simulink model "AutomaticWateringSystemProject"  (R2013b)
settings: Solver=ode3  SolverMode=SingleTasking  StartTime=0.0  StopTime=10.0  RelTol=1e-3
PreLoadFcn:
  | waijung.modelPreload; % Required for working with Waijung Blockset. Do not remove.
undefined symbols (not defined in the file): HSEOSC, Link, LQFP100, ST, STM32F407VG
libraries: stm32f4_io_lib x6, stm32f4_adc_lib x1, stm32f4_device_config_lib x1
(part 2 of 2)

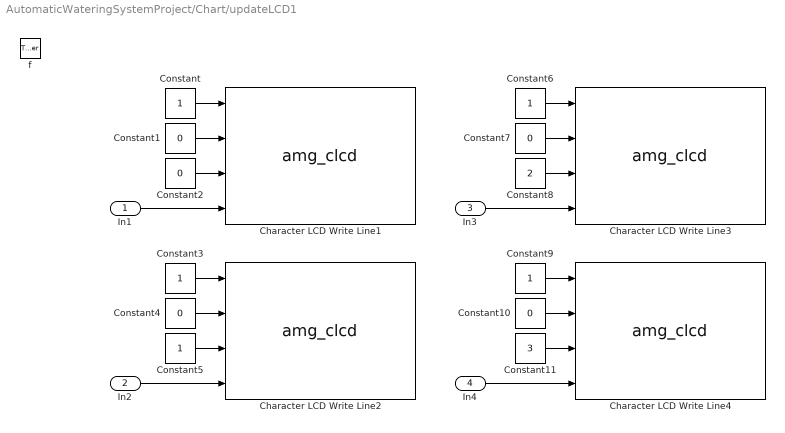
== system AutomaticWateringSystemProject/Chart/updateLCD1 ==
  In1 : Inport  OutDataTypeStr=uint8  PortDimensions=[1 16]
  In2 : Inport  Port=2  OutDataTypeStr=uint8  PortDimensions=[1 16]
  In3 : Inport  Port=3  OutDataTypeStr=uint8  PortDimensions=[1 16]
  In4 : Inport  Port=4  OutDataTypeStr=uint8  PortDimensions=[1 16]
  f : TriggerPort  TriggerType=function-call
      settings: CopyFcn=Stateflow.SLINSF.SimulinkMan.removeBlockPreDeleteFcn  PreDeleteFcn=Stateflow.SLINSF.SimulinkMan.unsafePredeleteFcn
  Character LCD Write Line1 : S-Function  FunctionName=amg_clcd  Parameters=module,configuration,inputtypearray,outputtypearray,confstr,sampletime,sampletimestr,blockid  EnableBusSupport=off  mask(amg_clcd){configuration=Transaction, module=1, model=amg CLCD Std, interface=4-bits, linecount=4, columncount=20, gpiotype=Push-pull, controlport=E, control_rs=15, control_rw=13, control_en=11, dataport=A, data0=7, data1=5, data2=3, data3=1, usestringbuffer=off, stringbuffer=<empty>, varname=, inputtypearray=[4 -1 -1 -1 -1], outputtypearray=[0], confstr=["4","4","20","PP","E","15","11","13","","A","","","","","7","5","3","1","0","","1","0","0","0","1","0","0","0","0","stm32f4"], sampletime=-1, sampletimestr=-1, blockid=ChartupdateLCD1CharacterLCDWriteLine1}
      mask prompts: model "LCD model:"; linecount "Number of lines:"; columncount "Number of columns:"; gpiotype "GPIO Output type:"; controlport "GPIO control port:"; control_rs "GPIO control pin, RS:"; control_rw "GPIO control pin, RW:"; control_en "GPIO control pin, EN:"; dataport "GPIO data D[7:4] port"; data0 "GPIO data pin, D4:"; data1 "GPIO data pin, D5:"; data2 "GPIO data pin, D6:"; data3 "GPIO data pin, D7:"; usestringbuffer "Use string buffer"; stringbuffer "String buffer"; varname "Variable name"; inputtypearray "Input type array"; outputtypearray "Output type array"; confstr "Configuration string"; sampletime "Sample time (sec)"; sampletimestr "Compiled sample time (sec) in string"
      mask help:
      | Note for cmd:
      | 1 - Clear specified LCD line display before write data to LCD.
      | Otherwise (e.g. 0) - Write data without clearing LCD Line.
      |
      | Position:
      | x = 0, First Character (from left to right)
      | y = 0, Top Line
      mask init:
      | amg_clcd_callback('init');
      mask Help: web(fullfile(waijungdocroot,'amg_clcd_write.htm'), '-browser')
      mask TypeOptions configuration: Setup | Transaction
      mask Callback configuration: amg_clcd_callback('configuration');
      mask TypeOptions module: 1 | 2 | 3 | 4
      mask TypeOptions model: amg CLCD Std
      mask TypeOptions interface: 4-bits
      mask TypeOptions gpiotype: Push-pull | Open-drain
      mask TypeOptions controlport: A | B | C | D | E | F | G | H | I
      mask TypeOptions control_rs: 0 | 1 | 2 | 3 | 4 | 5 | 6 | 7 | 8 | 9 | 10 | 11 | 12 | 13 | 14 | 15
      mask TypeOptions control_rw: 0 | 1 | 2 | 3 | 4 | 5 | 6 | 7 | 8 | 9 | 10 | 11 | 12 | 13 | 14 | 15
      mask TypeOptions control_en: 0 | 1 | 2 | 3 | 4 | 5 | 6 | 7 | 8 | 9 | 10 | 11 | 12 | 13 | 14 | 15
      mask TypeOptions dataport: A | B | C | D | E | F | G | H | I
      mask TypeOptions data0: 0 | 1 | 2 | 3 | 4 | 5 | 6 | 7 | 8 | 9 | 10 | 11 | 12 | 13 | 14 | 15
      mask TypeOptions data1: 0 | 1 | 2 | 3 | 4 | 5 | 6 | 7 | 8 | 9 | 10 | 11 | 12 | 13 | 14 | 15
      mask TypeOptions data2: 0 | 1 | 2 | 3 | 4 | 5 | 6 | 7 | 8 | 9 | 10 | 11 | 12 | 13 | 14 | 15
      mask TypeOptions data3: 0 | 1 | 2 | 3 | 4 | 5 | 6 | 7 | 8 | 9 | 10 | 11 | 12 | 13 | 14 | 15
      mask Callback usestringbuffer: amg_clcd_callback('usestringbuffer');
      mask TypeOptions stringbuffer: <empty>
      mask Callback varname: amg_clcd_callback('varname');
      mask Callback confstr: amg_clcd_callback('confstr');
      mask Callback sampletime: amg_clcd_callback('sampletime');
      mask Callback sampletimestr: amg_clcd_callback('sampletimestr');
      mask Callback blockid: amg_clcd_callback('blockid');
      mask Display: text(0.5, 0.5, 'Module: CLCD1 (Write)\nTs (sec): -1','ver','middle','hor','center');port_label('input', 1,'cmd');port_label('input', 2,'xpos');port_label('input', 3,'ypos');port_label('input', 4,'str');
  Character LCD Write Line2 : S-Function  FunctionName=amg_clcd  Parameters=module,configuration,inputtypearray,outputtypearray,confstr,sampletime,sampletimestr,blockid  EnableBusSupport=off  mask(amg_clcd){configuration=Transaction, module=1, model=amg CLCD Std, interface=4-bits, linecount=4, columncount=20, gpiotype=Push-pull, controlport=E, control_rs=15, control_rw=13, control_en=11, dataport=A, data0=7, data1=5, data2=3, data3=1, usestringbuffer=off, stringbuffer=<empty>, varname=, inputtypearray=[4 -1 -1 -1 -1], outputtypearray=[0], confstr=["4","4","20","PP","E","15","11","13","","A","","","","","7","5","3","1","0","","1","0","0","0","1","0","0","0","0","stm32f4"], sampletime=-1, sampletimestr=-1, blockid=ChartupdateLCD1CharacterLCDWriteLine2}
      mask prompts: model "LCD model:"; linecount "Number of lines:"; columncount "Number of columns:"; gpiotype "GPIO Output type:"; controlport "GPIO control port:"; control_rs "GPIO control pin, RS:"; control_rw "GPIO control pin, RW:"; control_en "GPIO control pin, EN:"; dataport "GPIO data D[7:4] port"; data0 "GPIO data pin, D4:"; data1 "GPIO data pin, D5:"; data2 "GPIO data pin, D6:"; data3 "GPIO data pin, D7:"; usestringbuffer "Use string buffer"; stringbuffer "String buffer"; varname "Variable name"; inputtypearray "Input type array"; outputtypearray "Output type array"; confstr "Configuration string"; sampletime "Sample time (sec)"; sampletimestr "Compiled sample time (sec) in string"
      mask help:
      | Note for cmd:
      | 1 - Clear specified LCD line display before write data to LCD.
      | Otherwise (e.g. 0) - Write data without clearing LCD Line.
      |
      | Position:
      | x = 0, First Character (from left to right)
      | y = 0, Top Line
      mask init:
      | amg_clcd_callback('init');
      mask Help: web(fullfile(waijungdocroot,'amg_clcd_write.htm'), '-browser')
      mask TypeOptions configuration: Setup | Transaction
      mask Callback configuration: amg_clcd_callback('configuration');
      mask TypeOptions module: 1 | 2 | 3 | 4
      mask TypeOptions model: amg CLCD Std
      mask TypeOptions interface: 4-bits
      mask TypeOptions gpiotype: Push-pull | Open-drain
      mask TypeOptions controlport: A | B | C | D | E | F | G | H | I
      mask TypeOptions control_rs: 0 | 1 | 2 | 3 | 4 | 5 | 6 | 7 | 8 | 9 | 10 | 11 | 12 | 13 | 14 | 15
      mask TypeOptions control_rw: 0 | 1 | 2 | 3 | 4 | 5 | 6 | 7 | 8 | 9 | 10 | 11 | 12 | 13 | 14 | 15
      mask TypeOptions control_en: 0 | 1 | 2 | 3 | 4 | 5 | 6 | 7 | 8 | 9 | 10 | 11 | 12 | 13 | 14 | 15
      mask TypeOptions dataport: A | B | C | D | E | F | G | H | I
      mask TypeOptions data0: 0 | 1 | 2 | 3 | 4 | 5 | 6 | 7 | 8 | 9 | 10 | 11 | 12 | 13 | 14 | 15
      mask TypeOptions data1: 0 | 1 | 2 | 3 | 4 | 5 | 6 | 7 | 8 | 9 | 10 | 11 | 12 | 13 | 14 | 15
      mask TypeOptions data2: 0 | 1 | 2 | 3 | 4 | 5 | 6 | 7 | 8 | 9 | 10 | 11 | 12 | 13 | 14 | 15
      mask TypeOptions data3: 0 | 1 | 2 | 3 | 4 | 5 | 6 | 7 | 8 | 9 | 10 | 11 | 12 | 13 | 14 | 15
      mask Callback usestringbuffer: amg_clcd_callback('usestringbuffer');
      mask TypeOptions stringbuffer: <empty>
      mask Callback varname: amg_clcd_callback('varname');
      mask Callback confstr: amg_clcd_callback('confstr');
      mask Callback sampletime: amg_clcd_callback('sampletime');
      mask Callback sampletimestr: amg_clcd_callback('sampletimestr');
      mask Callback blockid: amg_clcd_callback('blockid');
      mask Display: text(0.5, 0.5, 'Module: CLCD1 (Write)\nTs (sec): -1','ver','middle','hor','center');port_label('input', 1,'cmd');port_label('input', 2,'xpos');port_label('input', 3,'ypos');port_label('input', 4,'str');
  Character LCD Write Line3 : S-Function  FunctionName=amg_clcd  Parameters=module,configuration,inputtypearray,outputtypearray,confstr,sampletime,sampletimestr,blockid  EnableBusSupport=off  mask(amg_clcd){configuration=Transaction, module=1, model=amg CLCD Std, interface=4-bits, linecount=4, columncount=20, gpiotype=Push-pull, controlport=E, control_rs=15, control_rw=13, control_en=11, dataport=A, data0=7, data1=5, data2=3, data3=1, usestringbuffer=off, stringbuffer=<empty>, varname=, inputtypearray=[4 -1 -1 -1 -1], outputtypearray=[0], confstr=["4","4","20","PP","E","15","11","13","","A","","","","","7","5","3","1","0","","1","0","0","0","1","0","0","0","0","stm32f4"], sampletime=-1, sampletimestr=-1, blockid=ChartupdateLCD1CharacterLCDWriteLine3}
      mask prompts: model "LCD model:"; linecount "Number of lines:"; columncount "Number of columns:"; gpiotype "GPIO Output type:"; controlport "GPIO control port:"; control_rs "GPIO control pin, RS:"; control_rw "GPIO control pin, RW:"; control_en "GPIO control pin, EN:"; dataport "GPIO data D[7:4] port"; data0 "GPIO data pin, D4:"; data1 "GPIO data pin, D5:"; data2 "GPIO data pin, D6:"; data3 "GPIO data pin, D7:"; usestringbuffer "Use string buffer"; stringbuffer "String buffer"; varname "Variable name"; inputtypearray "Input type array"; outputtypearray "Output type array"; confstr "Configuration string"; sampletime "Sample time (sec)"; sampletimestr "Compiled sample time (sec) in string"
      mask help:
      | Note for cmd:
      | 1 - Clear specified LCD line display before write data to LCD.
      | Otherwise (e.g. 0) - Write data without clearing LCD Line.
      |
      | Position:
      | x = 0, First Character (from left to right)
      | y = 0, Top Line
      mask init:
      | amg_clcd_callback('init');
      mask Help: web(fullfile(waijungdocroot,'amg_clcd_write.htm'), '-browser')
      mask TypeOptions configuration: Setup | Transaction
      mask Callback configuration: amg_clcd_callback('configuration');
      mask TypeOptions module: 1 | 2 | 3 | 4
      mask TypeOptions model: amg CLCD Std
      mask TypeOptions interface: 4-bits
      mask TypeOptions gpiotype: Push-pull | Open-drain
      mask TypeOptions controlport: A | B | C | D | E | F | G | H | I
      mask TypeOptions control_rs: 0 | 1 | 2 | 3 | 4 | 5 | 6 | 7 | 8 | 9 | 10 | 11 | 12 | 13 | 14 | 15
      mask TypeOptions control_rw: 0 | 1 | 2 | 3 | 4 | 5 | 6 | 7 | 8 | 9 | 10 | 11 | 12 | 13 | 14 | 15
      mask TypeOptions control_en: 0 | 1 | 2 | 3 | 4 | 5 | 6 | 7 | 8 | 9 | 10 | 11 | 12 | 13 | 14 | 15
      mask TypeOptions dataport: A | B | C | D | E | F | G | H | I
      mask TypeOptions data0: 0 | 1 | 2 | 3 | 4 | 5 | 6 | 7 | 8 | 9 | 10 | 11 | 12 | 13 | 14 | 15
      mask TypeOptions data1: 0 | 1 | 2 | 3 | 4 | 5 | 6 | 7 | 8 | 9 | 10 | 11 | 12 | 13 | 14 | 15
      mask TypeOptions data2: 0 | 1 | 2 | 3 | 4 | 5 | 6 | 7 | 8 | 9 | 10 | 11 | 12 | 13 | 14 | 15
      mask TypeOptions data3: 0 | 1 | 2 | 3 | 4 | 5 | 6 | 7 | 8 | 9 | 10 | 11 | 12 | 13 | 14 | 15
      mask Callback usestringbuffer: amg_clcd_callback('usestringbuffer');
      mask TypeOptions stringbuffer: <empty>
      mask Callback varname: amg_clcd_callback('varname');
      mask Callback confstr: amg_clcd_callback('confstr');
      mask Callback sampletime: amg_clcd_callback('sampletime');
      mask Callback sampletimestr: amg_clcd_callback('sampletimestr');
      mask Callback blockid: amg_clcd_callback('blockid');
      mask Display: text(0.5, 0.5, 'Module: CLCD1 (Write)\nTs (sec): -1','ver','middle','hor','center');port_label('input', 1,'cmd');port_label('input', 2,'xpos');port_label('input', 3,'ypos');port_label('input', 4,'str');
  Character LCD Write Line4 : S-Function  FunctionName=amg_clcd  Parameters=module,configuration,inputtypearray,outputtypearray,confstr,sampletime,sampletimestr,blockid  EnableBusSupport=off  mask(amg_clcd){configuration=Transaction, module=1, model=amg CLCD Std, interface=4-bits, linecount=4, columncount=20, gpiotype=Push-pull, controlport=E, control_rs=15, control_rw=13, control_en=11, dataport=A, data0=7, data1=5, data2=3, data3=1, usestringbuffer=off, stringbuffer=<empty>, varname=, inputtypearray=[4 -1 -1 -1 -1], outputtypearray=[0], confstr=["4","4","20","PP","E","15","11","13","","A","","","","","7","5","3","1","0","","1","0","0","0","1","0","0","0","0","stm32f4"], sampletime=-1, sampletimestr=-1, blockid=ChartupdateLCD1CharacterLCDWriteLine4}
      mask prompts: model "LCD model:"; linecount "Number of lines:"; columncount "Number of columns:"; gpiotype "GPIO Output type:"; controlport "GPIO control port:"; control_rs "GPIO control pin, RS:"; control_rw "GPIO control pin, RW:"; control_en "GPIO control pin, EN:"; dataport "GPIO data D[7:4] port"; data0 "GPIO data pin, D4:"; data1 "GPIO data pin, D5:"; data2 "GPIO data pin, D6:"; data3 "GPIO data pin, D7:"; usestringbuffer "Use string buffer"; stringbuffer "String buffer"; varname "Variable name"; inputtypearray "Input type array"; outputtypearray "Output type array"; confstr "Configuration string"; sampletime "Sample time (sec)"; sampletimestr "Compiled sample time (sec) in string"
      mask help:
      | Note for cmd:
      | 1 - Clear specified LCD line display before write data to LCD.
      | Otherwise (e.g. 0) - Write data without clearing LCD Line.
      |
      | Position:
      | x = 0, First Character (from left to right)
      | y = 0, Top Line
      mask init:
      | amg_clcd_callback('init');
      mask Help: web(fullfile(waijungdocroot,'amg_clcd_write.htm'), '-browser')
      mask TypeOptions configuration: Setup | Transaction
      mask Callback configuration: amg_clcd_callback('configuration');
      mask TypeOptions module: 1 | 2 | 3 | 4
      mask TypeOptions model: amg CLCD Std
      mask TypeOptions interface: 4-bits
      mask TypeOptions gpiotype: Push-pull | Open-drain
      mask TypeOptions controlport: A | B | C | D | E | F | G | H | I
      mask TypeOptions control_rs: 0 | 1 | 2 | 3 | 4 | 5 | 6 | 7 | 8 | 9 | 10 | 11 | 12 | 13 | 14 | 15
      mask TypeOptions control_rw: 0 | 1 | 2 | 3 | 4 | 5 | 6 | 7 | 8 | 9 | 10 | 11 | 12 | 13 | 14 | 15
      mask TypeOptions control_en: 0 | 1 | 2 | 3 | 4 | 5 | 6 | 7 | 8 | 9 | 10 | 11 | 12 | 13 | 14 | 15
      mask TypeOptions dataport: A | B | C | D | E | F | G | H | I
      mask TypeOptions data0: 0 | 1 | 2 | 3 | 4 | 5 | 6 | 7 | 8 | 9 | 10 | 11 | 12 | 13 | 14 | 15
      mask TypeOptions data1: 0 | 1 | 2 | 3 | 4 | 5 | 6 | 7 | 8 | 9 | 10 | 11 | 12 | 13 | 14 | 15
      mask TypeOptions data2: 0 | 1 | 2 | 3 | 4 | 5 | 6 | 7 | 8 | 9 | 10 | 11 | 12 | 13 | 14 | 15
      mask TypeOptions data3: 0 | 1 | 2 | 3 | 4 | 5 | 6 | 7 | 8 | 9 | 10 | 11 | 12 | 13 | 14 | 15
      mask Callback usestringbuffer: amg_clcd_callback('usestringbuffer');
      mask TypeOptions stringbuffer: <empty>
      mask Callback varname: amg_clcd_callback('varname');
      mask Callback confstr: amg_clcd_callback('confstr');
      mask Callback sampletime: amg_clcd_callback('sampletime');
      mask Callback sampletimestr: amg_clcd_callback('sampletimestr');
      mask Callback blockid: amg_clcd_callback('blockid');
      mask Display: text(0.5, 0.5, 'Module: CLCD1 (Write)\nTs (sec): -1','ver','middle','hor','center');port_label('input', 1,'cmd');port_label('input', 2,'xpos');port_label('input', 3,'ypos');port_label('input', 4,'str');
  Constant{,3,5..6,9} (5 alike) : Constant
  Constant{1..2,4,7,10} (5 alike) : Constant  Value=0
  Constant11 : Constant  Value=3
  Constant8 : Constant  Value=2
  wires:
  In1/1 -> Character LCD Write Line1/4
  Constant/1 -> Character LCD Write Line1/1
  Constant1/1 -> Character LCD Write Line1/2
  Constant2/1 -> Character LCD Write Line1/3
  In2/1 -> Character LCD Write Line2/4
  Constant3/1 -> Character LCD Write Line2/1
  Constant4/1 -> Character LCD Write Line2/2
  Constant5/1 -> Character LCD Write Line2/3
  In3/1 -> Character LCD Write Line3/4
  Constant6/1 -> Character LCD Write Line3/1
  Constant7/1 -> Character LCD Write Line3/2
  Constant8/1 -> Character LCD Write Line3/3
  In4/1 -> Character LCD Write Line4/4
  Constant9/1 -> Character LCD Write Line4/1
  Constant10/1 -> Character LCD Write Line4/2
  Constant11/1 -> Character LCD Write Line4/3

== stateflow chart AutomaticWateringSystemProject/Chart ==
  state Initialization
  state NormalOperation
    state CheckKeyPress [parallel]
      settings: executionOrder=2
      state NoKeyPressed
        en: data = 0;
      state UpKeyPressed
        en: data = 1;
        state Short
        state Long
        (default) -> NormalOperation.CheckKeyPress.UpKeyPressed.Short : {UP_KEY_PRESSED;}
        NormalOperation.CheckKeyPress.UpKeyPressed.Short -> NormalOperation.CheckKeyPress.UpKeyPressed.Long : after(1,sec)
      state DownKeyPressed
        en: data = 1;
        state Short
        state Wait
        state Long
        note: {PRESS_DOWN_HOLD;}
        (default) -> NormalOperation.CheckKeyPress.DownKeyPressed.Short : {DOWN_KEY_PRESSED;}
        NormalOperation.CheckKeyPress.DownKeyPressed.Short -> NormalOperation.CheckKeyPress.DownKeyPressed.Long : after(1,sec)
        NormalOperation.CheckKeyPress.DownKeyPressed.Long -> Wait
      state OkKeyPressed
        en: data = 1;
        state Short
        (default) -> NormalOperation.CheckKeyPress.OkKeyPressed.Short : {OK_KEY_PRESSED;}
      (default) -> NoKeyPressed
      NoKeyPressed -> UpKeyPressed [order 1] : [up_key == 1]
      UpKeyPressed -> NoKeyPressed : [up_key == 0]
      NoKeyPressed -> DownKeyPressed [order 2] : [down_key == 1]
      DownKeyPressed -> NoKeyPressed : [down_key == 0]
      NoKeyPressed -> OkKeyPressed [order 3] : [ok_key == 1]
      OkKeyPressed -> NoKeyPressed : [ok_key == 0]
    state MenuDisplay [parallel]
      settings: executionOrder=1
      state Screen1
        en: lcd_line1 = setLcdLine1(1);
        en: lcd_line2 = setLcdLine2(1);
        en: lcd_line3 = setLcdLine3(1);
        en: lcd_line4 = setLcdLine4(1);
        en: updateLCD1(lcd_line1,lcd_line2,lcd_line3,lcd_line4);
      state Screen2
        en: lcd_line1 = setLcdLine1(2);
        en: lcd_line2 = setLcdLine2(2);
        en: lcd_line3 = setLcdLine3(2);
        en: lcd_line4 = setLcdLine4(0);
        en: updateLCD1(lcd_line1,lcd_line2,lcd_line3,lcd_line4);
      state Screen3
        en: lcd_line1 = setLcdLine1(3);
        en: updateDate();
        en: updateStartHour();
        en: updateStartMinute();
        en: updateLCD1(lcd_line1,lcd_line2,lcd_line3,lcd_line4);
      state Screen31
        en: lcd_line1 = setLcdLine1(3);
        en: updateDate();
        en: updateStopHour();
        en: updateStopMinute();
        en: updateLCD1(lcd_line1,lcd_line2,lcd_line3,lcd_line4);
      state Screen32
        en: lcd_line1 = setLcdLine1(4);
        en: updateNPK46();
        en: updateNPK15();
        en: updateMois();
        en: updateLCD1(lcd_line1,lcd_line2,lcd_line3,lcd_line4);
      state Screen5
        en: lcd_line1 = setLcdLine1(5);
        en: updateVALVEbtn();
        en: updateNPK46btn();
        en: updateNPK15btn();
        en: updateLCD1(lcd_line1,lcd_line2,lcd_line3,lcd_line4);
      state Screen21
        en: lcd_line1 = setLcdLine1(2);
        en: lcd_line2 = setLcdLine2(3);
        en: lcd_line3 = setLcdLine3(3);
        en: lcd_line4 = setLcdLine4(0);
        en: updateLCD1(lcd_line1,lcd_line2,lcd_line3,lcd_line4);
      Screen3 -> Screen3 [order 2] : after(1.5,sec)
      (default) -> Screen1
      Screen1 -> Screen2 : OK_KEY_PRESSED
      Screen2 -> Screen3 [order 2] : OK_KEY_PRESSED
      Screen3 -> Screen2 [order 1] : [in(CheckKeyPress.DownKeyPressed.Long)]
      Screen2 -> Screen21 [order 1] : DOWN_KEY_PRESSED
      Screen21 -> Screen2 [order 1] : UP_KEY_PRESSED
      Screen32 -> Screen2 [order 3] : [in(CheckKeyPress.DownKeyPressed.Long)]
      Screen21 -> Screen1 [order 3] : [in(CheckKeyPress.DownKeyPressed.Long)]
      Screen3 -> Screen31 [order 3] : DOWN_KEY_PRESSED
      Screen31 -> Screen3 [order 2] : UP_KEY_PRESSED
      Screen31 -> Screen31 [order 3] : after(1.5,sec)
      Screen31 -> Screen32 [order 1] : DOWN_KEY_PRESSED
      Screen32 -> Screen31 [order 1] : UP_KEY_PRESSED
      Screen32 -> Screen32 [order 2] : after(1.5,sec)
      Screen5 -> Screen5 [order 2] : after(1.5,sec)
      Screen5 -> Screen21 [order 1] : [in(CheckKeyPress.DownKeyPressed.Long)]
      Screen21 -> Screen5 [order 2] : OK_KEY_PRESSED
  state updateLCD1(In1,In2,In3,In4) [function]
  (default) -> Initialization
  Initialization -> NormalOperation
  data: option function_input double; outstr function_output uint8 size=[1 16]; option function_input double; outstr function_output uint8 size=[1 16]; option function_input double; outstr function_output uint8 size=[1 16]; option function_input double; outstr function_output uint8 size=[1 16]; In1 function_input uint8 size=[1 16]; In2 function_input uint8 size=[1 16]; In3 function_input uint8 size=[1 16]; In4 function_input uint8 size=[1 16]; ok_key input; up_key input; down_key input; data output double =0; lcd_line1 local uint8 size=[1 16]; lcd_line2 local uint8 size=[1 16]; lcd_line3 local uint8 size=[1 16]; lcd_line4 local uint8 size=[1 16]; Mois input double; Date input double; StartHour input double; StartMinute input double; StopHour input double; StopMinute input double; NPK46 input double; NPK15 input double; VALVEbtn input double; NPK46btn input double; NPK15btn input double
  events: triger input RISING_EDGE_EVENT; UP_KEY_PRESSED local FUNCTION_CALL_EVENT; OK_KEY_PRESSED local FUNCTION_CALL_EVENT; DOWN_KEY_PRESSED local FUNCTION_CALL_EVENT; PRESS_DOWN_HOLD local FUNCTION_CALL_EVENT
  function outstr = setLcdLine1(option):
    | function outstr = setLcdLine1(option)
    | 
    | switch option
    |     case 0             %0123456789ABCDEF
    |         outstr = uint8('                ');
    |     case 1  
    |         outstr = uint8('   AUTOMATIC    ');
    |     case 2 
    |         outstr = uint8(' WATERING STATUS');
    |     case 3 
    |         outstr = uint8('   DATE & TIME  ');
    |     case 4 
    |         outstr = uint8('   FERTILIZER   ');
    |     case 5 
    |         outstr = uint8('     MANUAL     ');
    |     otherwise
    |         outstr = uint8('                ');
    | end
  function outstr = setLcdLine2(option):
    | function outstr = setLcdLine2(option)
    | 
    | switch option
    |     case 0             %0123456789ABCDEF
    |         outstr = uint8('                ');
    |     case 1  
    |         outstr = uint8(' WATERING SYSTEM');
    |     case 2 
    |         outstr = uint8('>AUTOMATIC      ');
    |     case 3
    |         outstr = uint8(' AUTOMATIC      ');
    |     case 4
    |         outstr = uint8('DATE:           ');
    |     case 5
    |         outstr = uint8('NPK46:          ');
    |     case 6
    |         outstr = uint8('VALVE:          ');
    |     otherwise
    |         outstr = uint8('                ');
    | end
  function updateDate:
    | function updateDate
    | coder.ceval('sprintf',coder.ref(lcd_line2), ['DATE: %02.0f          '],Date);
  function updateStartHour:
    | function updateStartHour
    | coder.ceval('sprintf',coder.ref(lcd_line3), ['START TIME: %02.0fHH  '],StartHour);
  function updateStartMinute:
    | function updateStartMinute
    | coder.ceval('sprintf',coder.ref(lcd_line4), ['          : %02.0fMM  '],StartMinute);
  function updateStopHour:
    | function updateStopHour
    | coder.ceval('sprintf',coder.ref(lcd_line3), ['STOP TIME: %02.0fHH   '],StopHour);
  function updateStopMinute:
    | function updateStopMinute
    | coder.ceval('sprintf',coder.ref(lcd_line4), ['         : %02.0fMM   '],StopMinute);
  function updateNPK46:
    | function updateNPK46
    | coder.ceval('sprintf',coder.ref(lcd_line2), ['NPK46: %02.0f Sec     '],NPK46);
  function updateNPK15:
    | function updateNPK15
    | coder.ceval('sprintf',coder.ref(lcd_line3), ['NPK15: %02.0f Sec     '],NPK15);
  function updateMois:
    | function updateMois
    | coder.ceval('sprintf',coder.ref(lcd_line4), ['MOISTURE: %04.1f %%   '],Mois);
  function updateVALVEbtn:
    | function updateVALVEbtn
    |     switch VALVEbtn
    |         case 0
    |         coder.ceval('sprintf',coder.ref(lcd_line2), ['VALVE: OFF            '],VALVEbtn);
    |         case 1
    |         coder.ceval('sprintf',coder.ref(lcd_line2), ['VALVE: ON             '],VALVEbtn);     
    |     end
  function updateNPK46btn:
    | function updateNPK46btn
    |     switch NPK46btn
    |         case 0
    |         coder.ceval('sprintf',coder.ref(lcd_line3), ['NPK46: OFF            '],NPK46btn);
    |         case 1
    |         coder.ceval('sprintf',coder.ref(lcd_line3), ['NPK46: ON             '],NPK46btn);     
    |     end
  function updateNPK15btn:
    | function updateNPK15btn
    |     switch NPK15btn
    |         case 0
    |         coder.ceval('sprintf',coder.ref(lcd_line4), ['NPK15: OFF            '],NPK15btn);
    |         case 1
    |         coder.ceval('sprintf',coder.ref(lcd_line4), ['NPK15: ON             '],NPK15btn);     
    |     end
  function outstr = setLcdLine3(option):
    | function outstr = setLcdLine3(option)
    | 
    | switch option
    |     case 0             %0123456789ABCDEF
    |         outstr = uint8('                ');
    |     case 1  
    |         outstr = uint8('SENEE & NATHAPOP');
    |     case 2 
    |         outstr = uint8(' MANUAL         ');
    |     case 3 
    |         outstr = uint8('>MANUAL         ');
    |     case 4 
    |         outstr = uint8('START TIME:     ');
    |     case 5 
    |         outstr = uint8('NPK15:          ');
    |     case 6 
    |         outstr = uint8('NPK46:          ');
    |     case 7
    |         outstr = uint8('MOISTURE=    %  ');
    |     otherwise
    |         outstr = uint8('                ');
    | end
  function outstr = setLcdLine4(option):
    | function outstr = setLcdLine4(option)
    | 
    | switch option
    |     case 0             %0123456789ABCDEF
    |         outstr = uint8('                ');
    |     case 1  
    |         outstr = uint8(' EE3705 SEC:641 ');
    |     case 2 
    |         outstr = uint8('STOP TIME:      ');
    |     case 3 
    |         outstr = uint8('SOIL MOISTURE:  ');
    |     case 4 
    |         outstr = uint8('NPK15:          ');   
    |     otherwise
    |         outstr = uint8('                ');
    | end
